simulink model "engine_core"  (R2026a)
settings: Solver=VariableStepAuto  StopTime=300
undefined symbols (not defined in the file): engine
settings Model: LastModifiedBy=GOD

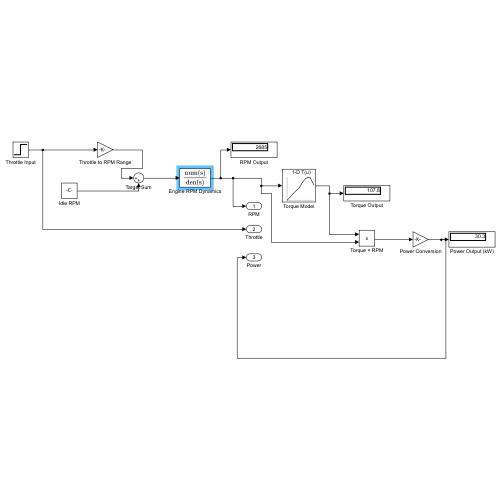
[thumbnail: Simulink's stored preview of the top-level diagram]
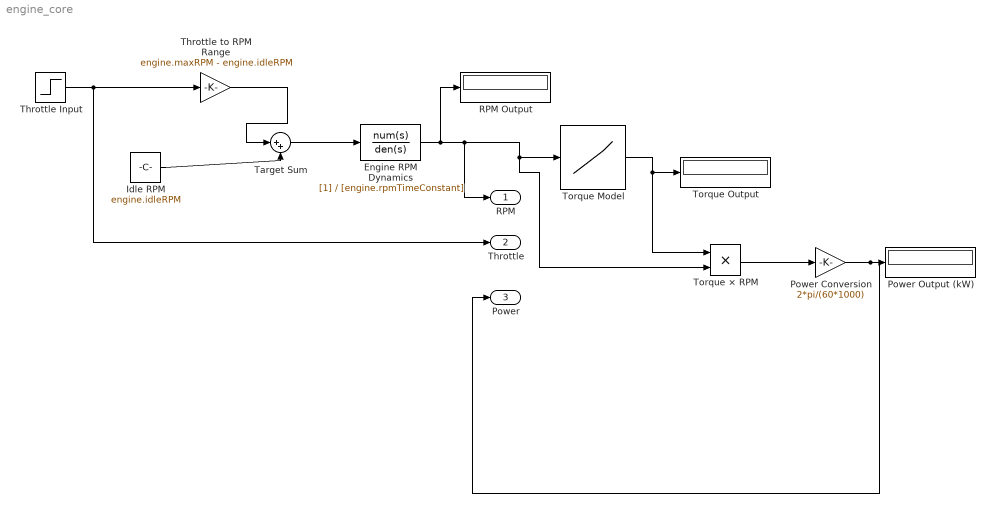
== system engine_core ==
  Engine RPM Dynamics : TransferFcn  Denominator=[engine.rpmTimeConstant]
  Idle RPM : Constant  Value=engine.idleRPM
  Power Conversion : Gain  Gain=2*pi/(60*1000)
  Power Output (kW) : Display
  RPM Output : Display
  Target Sum : Sum  Inputs=|++
  Throttle Input : Step  Time=0  FinalValue=0.9  SampleTime=0
  Throttle to RPM Range : Gain  Gain=engine.maxRPM - engine.idleRPM
  "Torque Model " : Lookup_n-D  NumberOfTableDimensions=1  BreakpointsForDimension1=[1500 2500 3500 4000 4500 4900 5200 5500 5800]  Table=[90 105 120 132 140 144 142 135 126]  InternalRulePriority=Speed  RndMeth=Simplest
  Torque Output : Display
  Torque × RPM : Product
  RPM : Outport
  Throttle : Outport  Port=2
  Power : Outport  Port=3
  wires:
  Throttle Input/1 -> Throttle/1, Throttle to RPM Range/1
  Throttle to RPM Range/1 -> Target Sum/1
  Idle RPM/1 -> Target Sum/2
  Target Sum/1 -> Engine RPM Dynamics/1
  Engine RPM Dynamics/1 -> RPM/1, Torque × RPM/2, "Torque Model "/1, RPM Output/1
  "Torque Model "/1 -> Torque × RPM/1, Torque Output/1
  Torque × RPM/1 -> Power Conversion/1
  Power Conversion/1 -> Power/1, Power Output (kW)/1
